simulink model "gm_untitled_vnl"  (R2022a)
settings: Solver=FixedStepDiscrete  StartTime=0.0  StopTime=2000  RelTol=1e-3
libraries: dspsigops x6, simulink x3, hdlsllib x2, simulink_need_slupdate x2
Description:
  | Symmetric FIR Filter
  | This example shows how to use HDL Coder(TM) to check, generate,
  | and verify HDL for a fixed-point symmetric FIR filter.
settings Model: Creator=okoko  LastModifiedBy=okoko
settings SolverCC: AlgebraicLoopSolver=TrustRegion
settings DataIOCC: LimitDataPoints=on  SaveOutput=off  SignalLogging=off  SaveTime=off  SignalLoggingName=logsOut
settings OptimizationCC: BlockReduction=off  BooleanDataType=off  ConditionallyExecuteInputs=off  DefaultParameterBehavior=Inlined  InlineInvariantSignals=on  ExpressionDepthLimit=2147483647  InitFltsAndDblsToZero=on  LifeSpan=inf  BufferReusableBoundary=off
settings DebuggingCC: AlgebraicLoopMsg=error  SaveWithParameterizedLinksMsg=none  UnderspecifiedInitializationDetection=Classic  MergeDetectMultiDrivingBlocksExec=none  CheckExecutionContextPreStartOutputMsg=on  SignalResolutionControl=TryResolveAllWithWarning  InheritedTsInSrcMsg=none  MultiTaskDSMMsg=warning  MultiTaskCondExecSysMsg=none  SingleTaskRateTransMsg=error  IntegerOverflowMsg=none  ParameterPrecisionLossMsg=none  FcnCallInpInsideContextMsg=warning  UnconnectedInputMsg=warning  UnconnectedOutputMsg=warning  UnconnectedLineMsg=warning  BusObjectLabelMismatch=none  AllowSymbolicDim=off  StateNameClashWarn=warning  StrictBusMsg=ErrorOnBusTreatedAsVector  SFUnexpectedBacktrackingDiag=warning  SFNoUnconditionalDefaultTransitionDiag=warning  SFExecutionAtInitializationDiag=none  SFMachineParentedDataDiag=warning  IntegerSaturationMsg=none  ArithmeticOperatorsInVariantConditions=warning
settings HardwareCC: ProdBitPerPointer=32  ProdBitPerSizeT=32  ProdBitPerPtrDiffT=32  ProdLargestAtomicFloat=None  ProdIntDivRoundTo=Undefined  ProdEndianess=Unspecified  ProdWordSize=32  ProdHWDeviceType=ASIC/FPGA->ASIC/FPGA  TargetUnknown=on  ProdEqTarget=off
settings SFSimCC: SimUseLocalCustomCode=off  CustomCodeUndefinedFunction=UseInterfaceOnly
settings RTWCC: RTWUseLocalCustomCode=off
settings CodeAppCC: StateflowObjectComments=on
settings GRTTargetCC: TargetFcnLib=ansi_tfl_tmw.mat  TargetLangStandard=C89/C90 (ANSI)  CombineOutputUpdateFcns=off  GRTInterface=on
settings ConfigComp: CovScope=ReferencedModels  CovMetricSettings=dw  CovSaveCumulativeToWorkspaceVar=on  CovSaveSingleToWorkspaceVar=on  CovExternalEMLEnable=off  CovSFcnEnable=off

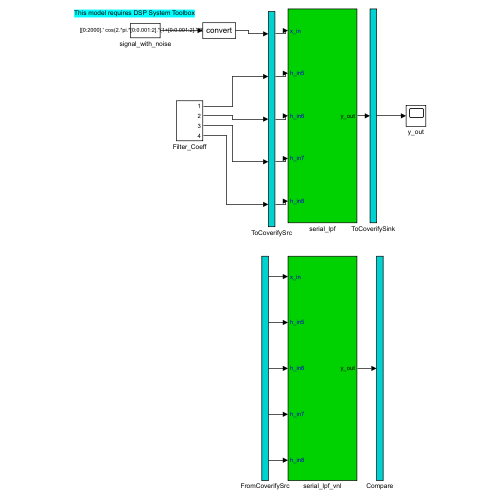
[thumbnail: Simulink's stored preview of the top-level diagram]
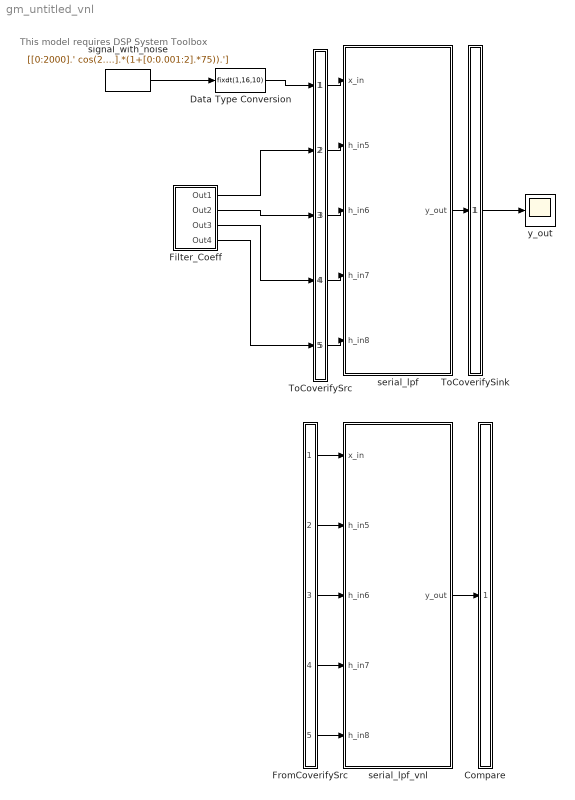
== system gm_untitled_vnl ==
  note: This model requires DSP System Toolbox
  Compare : Subsystem
      mask Display: disp('')
  Data Type Conversion : DataTypeConversion  OutDataTypeStr=fixdt(1,16,10)  SaturateOnIntegerOverflow=off  RndMeth=Floor
  Filter_Coeff : Subsystem
  FromCoverifySrc : Subsystem
      mask Display: disp('')
  ToCoverifySink : Subsystem
      mask Display: disp('')
  ToCoverifySrc : Subsystem
      mask Display: disp('')
  serial_lpf : Subsystem
  serial_lpf_vnl : Subsystem
  signal_with_noise : FromWorkspace  VariableName=[[0:2000].' cos(2.*pi.*[0:0.001:2].*(1+[0:0.001:2].*75)).']  SampleTime=1  OutputAfterFinalValue=Setting to zero
  y_out : Scope
  wires:
  signal_with_noise/1 -> Data Type Conversion/1
  ToCoverifySrc/1(out1) -> serial_lpf/1(x_in)
  ToCoverifySrc/2(out2) -> serial_lpf/2(h_in5)
  ToCoverifySrc/3(out3) -> serial_lpf/3(h_in6)
  ToCoverifySrc/4(out4) -> serial_lpf/4(h_in7)
  ToCoverifySrc/5(out5) -> serial_lpf/5(h_in8)
  serial_lpf/1(y_out) -> ToCoverifySink/1(in1)
  Data Type Conversion/1 -> ToCoverifySrc/1(in1)
  Filter_Coeff/1(Out1) -> ToCoverifySrc/2(in2)
  Filter_Coeff/2(Out2) -> ToCoverifySrc/3(in3)
  Filter_Coeff/3(Out3) -> ToCoverifySrc/4(in4)
  Filter_Coeff/4(Out4) -> ToCoverifySrc/5(in5)
  ToCoverifySink/1(out1) -> y_out/1
  FromCoverifySrc/1(out1) -> serial_lpf_vnl/1(x_in)
  FromCoverifySrc/2(out2) -> serial_lpf_vnl/2(h_in5)
  FromCoverifySrc/3(out3) -> serial_lpf_vnl/3(h_in6)
  FromCoverifySrc/4(out4) -> serial_lpf_vnl/4(h_in7)
  FromCoverifySrc/5(out5) -> serial_lpf_vnl/5(h_in8)
  serial_lpf_vnl/1(y_out) -> Compare/1(in1)

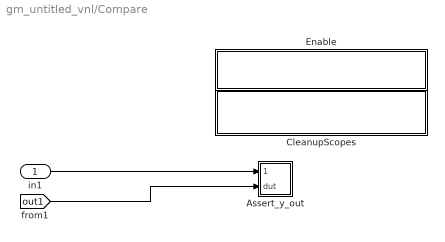
== system gm_untitled_vnl/Compare ==
  in1 : Inport
  Assert_y_out : Subsystem
  CleanupScopes : Subsystem
      settings: OpenFcn=|
      | blkName = gcb; %self block
      | idx = regexp(blkName, '/CleanupScopes$', 'once');
      | blkParent = blkName(1:idx-1);
      | blks=find_system(blkParent, 'LookUnderMasks', 'all','blocktype', 'Scope');
      | for itr = 1:length(blks)
      | 	 hScopeCfg = get_param(blks{itr},'ScopeConfiguration');
      | 	 hScopeCfg.Visible = ~ hScopeCfg.Visible;
      | end
      | drawnow;
      mask Display: fprintf(message('hdlcoder:cosim:vnl_dblclick').getString());
  Enable : Subsystem
      settings: OpenFcn=|
      | blkName = gcb;
      | idx = regexp(blkName, '/Enable$', 'once');
      | blkParent = blkName(1:idx-1);
      | blks=find_system(blkParent, 'LookUnderMasks', 'all','blocktype', 'Assertion');
      | e = get_param(blks{1}, 'Enabled');
      | if strcmp(e, 'on'), f= 'off';, else, f = 'on';, end
      | for ii=1:length(blks), set_param(blks{ii}, 'Enabled', f);, end
      | set_param(gcb, 'MaskDisplay',['fprintf(message(''hdlcoder:cosim:vnl_dblclick_assertions'',','''',upper(e),'''',').getString())']);
      mask Display: fprintf(message('hdlcoder:cosim:vnl_dblclick_assertions','OFF').getString());
  wires:
  in1/1 -> Assert_y_out/1(cosim)
  [out1] -> Assert_y_out/2(dut)

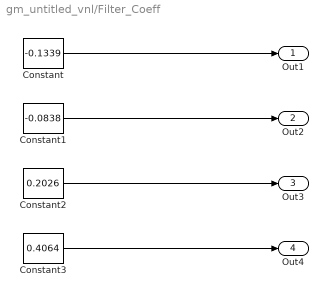
== system gm_untitled_vnl/Filter_Coeff ==
  Constant : Constant  Value=-0.1339  OutDataTypeStr=fixdt(1,16,10)  SampleTime=1
  Constant1 : Constant  Value=-0.0838  OutDataTypeStr=fixdt(1,16,10)  SampleTime=1
  Constant2 : Constant  Value=0.2026  OutDataTypeStr=fixdt(1,16,10)  SampleTime=1
  Constant3 : Constant  Value=0.4064  OutDataTypeStr=fixdt(1,16,10)  SampleTime=1
  Out1 : Outport  VectorParamsAs1DForOutWhenUnconnected=off
  Out2 : Outport  Port=2  VectorParamsAs1DForOutWhenUnconnected=off
  Out3 : Outport  Port=3  VectorParamsAs1DForOutWhenUnconnected=off
  Out4 : Outport  Port=4  VectorParamsAs1DForOutWhenUnconnected=off
  wires:
  Constant1/1 -> Out2/1
  Constant3/1 -> Out4/1
  Constant2/1 -> Out3/1
  Constant/1 -> Out1/1

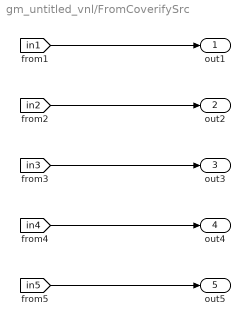
== system gm_untitled_vnl/FromCoverifySrc ==
  out1 : Outport
  out2 : Outport  Port=2
  out3 : Outport  Port=3
  out4 : Outport  Port=4
  out5 : Outport  Port=5
  wires:
  [in1] -> out1/1
  [in2] -> out2/1
  [in3] -> out3/1
  [in4] -> out4/1
  [in5] -> out5/1

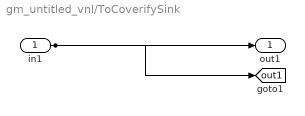
== system gm_untitled_vnl/ToCoverifySink ==
  in1 : Inport
  out1 : Outport
  tag scope: out1=global
  wires:
  in1/1 -> out1/1, [out1]

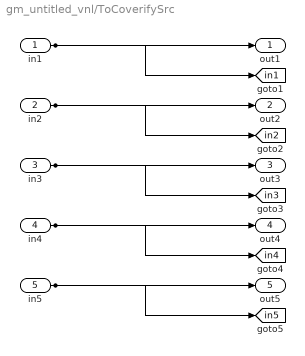
== system gm_untitled_vnl/ToCoverifySrc ==
  in1 : Inport
  in2 : Inport  Port=2
  in3 : Inport  Port=3
  in4 : Inport  Port=4
  in5 : Inport  Port=5
  out1 : Outport
  out2 : Outport  Port=2
  out3 : Outport  Port=3
  out4 : Outport  Port=4
  out5 : Outport  Port=5
  tag scope: in1=global, in2=global, in3=global, in4=global, in5=global
  wires:
  in1/1 -> out1/1, [in1]
  in2/1 -> out2/1, [in2]
  in3/1 -> out3/1, [in3]
  in4/1 -> out4/1, [in4]
  in5/1 -> out5/1, [in5]

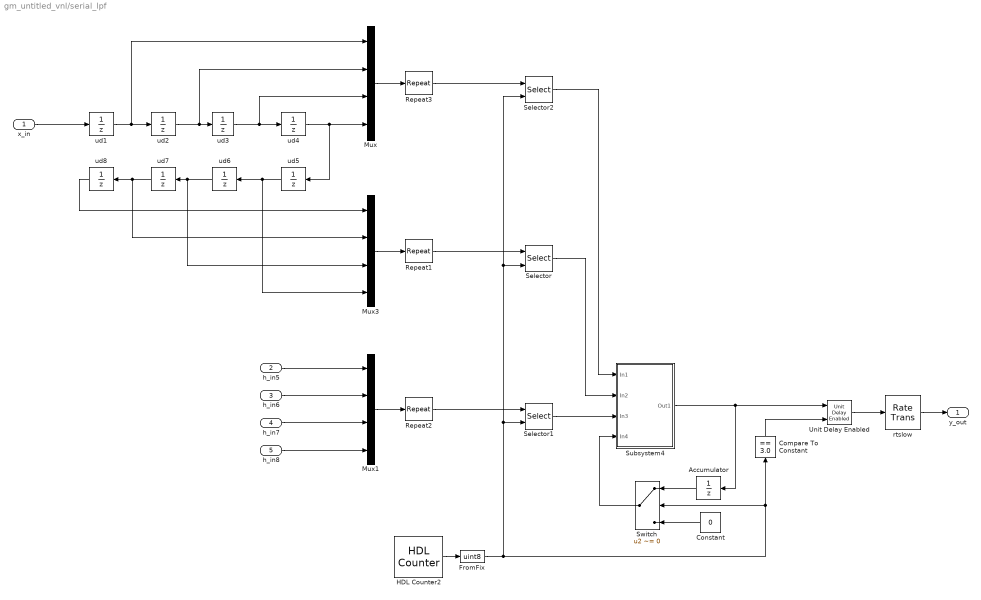
== system gm_untitled_vnl/serial_lpf ==
  x_in : Inport  SampleTime=1
  h_in5 : Inport  Port=2
  h_in6 : Inport  Port=3
  h_in7 : Inport  Port=4
  h_in8 : Inport  Port=5
  Accumulator : UnitDelay  SampleTime=-1  HasFrameUpgradeWarning=on
  Compare To Constant : simulink/Logic and Bit Operations/Compare To Constant  relop===  const=3.0  OutDataTypeStr=boolean
  Constant : Constant  Value=0  OutDataTypeStr=Inherit: Inherit via back propagation  SampleTime=-1
  FromFix : DataTypeConversion  OutDataTypeStr=uint8  SaturateOnIntegerOverflow=off  RndMeth=Floor
  HDL Counter2 : hdlsllib/Sources/HDL Counter  CountType=Count limited  CountInit=0  CountStep=1  CountMax=3  CountFromType=Initial value  CountFrom=0  CountResetPort=off  CountLoadPort=off  CountEnbPort=off  CountDirPort=off  CountHitOutputPort=off  CountDataType=Unsigned  CountWordLen=2  CountFracLen=0  CountSampTime=-1
  Mux : Mux
  Mux1 : Mux
  Mux3 : Mux
  Repeat1 : dspsigops/Repeat  N=4  RateOptions=Allow multirate processing  ic=0  mode=Unused parameter value
  Repeat2 : dspsigops/Repeat  N=4  RateOptions=Allow multirate processing  ic=0  mode=Unused parameter value
  Repeat3 : dspsigops/Repeat  N=4  RateOptions=Allow multirate processing  ic=0  mode=Unused parameter value
  Selector : Selector  IndexMode=Zero-based  InputPortWidth=4  IndexOptions=Index vector (port)  Indices=[1 3]  OutputSizes=1
  Selector1 : Selector  IndexMode=Zero-based  InputPortWidth=4  IndexOptions=Index vector (port)  Indices=[1 3]  OutputSizes=1
  Selector2 : Selector  IndexMode=Zero-based  InputPortWidth=4  IndexOptions=Index vector (port)  Indices=[1 3]  OutputSizes=1
  Subsystem4 : Subsystem  TreatAsAtomicUnit=on
  Switch : Switch  Criteria=u2 ~= 0  OutDataTypeStr=fixdt(1,35,20)  SaturateOnIntegerOverflow=off  InputSameDT=off
  Unit Delay Enabled : simulink_need_slupdate/Unit Delay Enabled  vinit=0.0  tsamp=-1
      settings: SourceProductBaseCode=SL
  rtslow : RateTransition
  ud{1..8} (8 alike) : UnitDelay  SampleTime=-1  HasFrameUpgradeWarning=on
  y_out : Outport  SampleTime=1  VectorParamsAs1DForOutWhenUnconnected=off
  wires:
  Selector/1 -> Subsystem4/2(In2)
  Mux/1 -> Repeat3/1
  Repeat1/1 -> Selector/1
  Subsystem4/1(Out1) -> Accumulator/1, Unit Delay Enabled/1
  x_in/1 -> ud1/1
  ud7/1 -> Mux3/2, ud8/1
  h_in5/1 -> Mux1/1
  h_in6/1 -> Mux1/2
  h_in7/1 -> Mux1/3
  h_in8/1 -> Mux1/4
  HDL Counter2/1 -> FromFix/1
  Mux1/1 -> Repeat2/1
  Selector1/1 -> Subsystem4/3(In3)
  Selector2/1 -> Subsystem4/1(In1)
  Mux3/1 -> Repeat1/1
  Repeat3/1 -> Selector2/1
  Repeat2/1 -> Selector1/1
  rtslow/1 -> y_out/1
  Unit Delay Enabled/1 -> rtslow/1
  Accumulator/1 -> Switch/1
  Constant/1 -> Switch/3
  Switch/1 -> Subsystem4/4(In4)
  Compare To Constant/1 -> Unit Delay Enabled/2
  ud1/1 -> Mux/1, ud2/1
  ud2/1 -> Mux/2, ud3/1
  ud3/1 -> Mux/3, ud4/1
  ud4/1 -> Mux/4, ud5/1
  ud5/1 -> Mux3/4, ud6/1
  ud6/1 -> Mux3/3, ud7/1
  ud8/1 -> Mux3/1
  FromFix/1 -> Selector1/2, Selector/2, Selector2/2, Switch/2, Compare To Constant/1

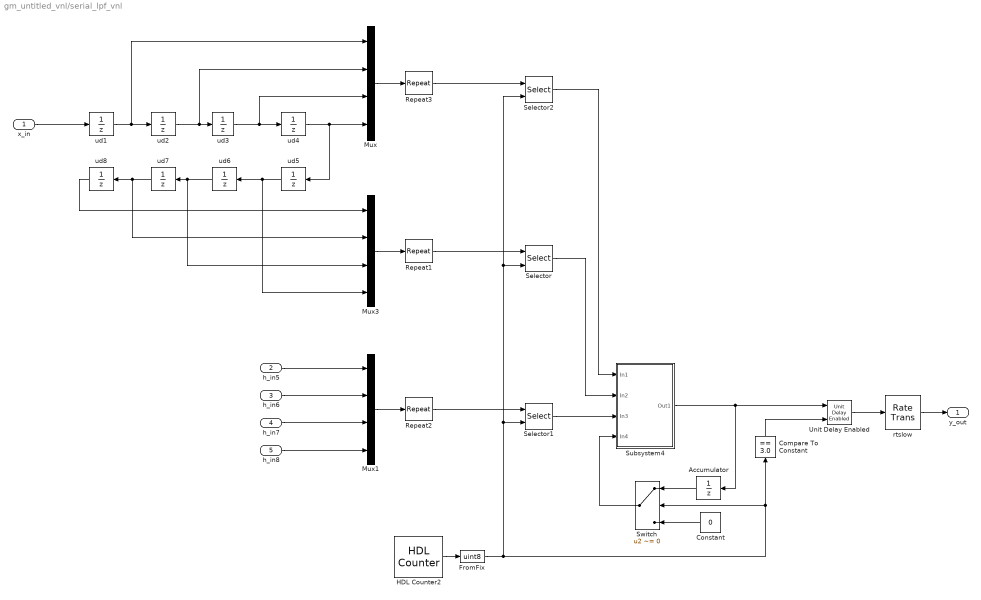
== system gm_untitled_vnl/serial_lpf_vnl ==
  x_in : Inport  SampleTime=1
  h_in5 : Inport  Port=2
  h_in6 : Inport  Port=3
  h_in7 : Inport  Port=4
  h_in8 : Inport  Port=5
  Accumulator : UnitDelay  SampleTime=-1  HasFrameUpgradeWarning=on
  Compare To Constant : simulink/Logic and Bit Operations/Compare To Constant  relop===  const=3.0  OutDataTypeStr=boolean
  Constant : Constant  Value=0  OutDataTypeStr=Inherit: Inherit via back propagation  SampleTime=-1
  FromFix : DataTypeConversion  OutDataTypeStr=uint8  SaturateOnIntegerOverflow=off  RndMeth=Floor
  HDL Counter2 : hdlsllib/Sources/HDL Counter  CountType=Count limited  CountInit=0  CountStep=1  CountMax=3  CountFromType=Initial value  CountFrom=0  CountResetPort=off  CountLoadPort=off  CountEnbPort=off  CountDirPort=off  CountHitOutputPort=off  CountDataType=Unsigned  CountWordLen=2  CountFracLen=0  CountSampTime=-1
  Mux : Mux
  Mux1 : Mux
  Mux3 : Mux
  Repeat1 : dspsigops/Repeat  N=4  RateOptions=Allow multirate processing  ic=0  mode=Unused parameter value
  Repeat2 : dspsigops/Repeat  N=4  RateOptions=Allow multirate processing  ic=0  mode=Unused parameter value
  Repeat3 : dspsigops/Repeat  N=4  RateOptions=Allow multirate processing  ic=0  mode=Unused parameter value
  Selector : Selector  IndexMode=Zero-based  InputPortWidth=4  IndexOptions=Index vector (port)  Indices=[1 3]  OutputSizes=1
  Selector1 : Selector  IndexMode=Zero-based  InputPortWidth=4  IndexOptions=Index vector (port)  Indices=[1 3]  OutputSizes=1
  Selector2 : Selector  IndexMode=Zero-based  InputPortWidth=4  IndexOptions=Index vector (port)  Indices=[1 3]  OutputSizes=1
  Subsystem4 : Subsystem  TreatAsAtomicUnit=on
  Switch : Switch  Criteria=u2 ~= 0  OutDataTypeStr=fixdt(1,35,20)  SaturateOnIntegerOverflow=off  InputSameDT=off
  Unit Delay Enabled : simulink_need_slupdate/Unit Delay Enabled  vinit=0.0  tsamp=-1
      settings: SourceProductBaseCode=SL
  rtslow : RateTransition
  ud{1..8} (8 alike) : UnitDelay  SampleTime=-1  HasFrameUpgradeWarning=on
  y_out : Outport  SampleTime=1  VectorParamsAs1DForOutWhenUnconnected=off
  wires:
  FromFix/1 -> Compare To Constant/1, Switch/2, Selector2/2, Selector/2, Selector1/2
  ud8/1 -> Mux3/1
  ud6/1 -> ud7/1, Mux3/3
  ud5/1 -> ud6/1, Mux3/4
  ud4/1 -> ud5/1, Mux/4
  ud3/1 -> ud4/1, Mux/3
  ud2/1 -> ud3/1, Mux/2
  ud1/1 -> ud2/1, Mux/1
  Compare To Constant/1 -> Unit Delay Enabled/2
  Switch/1 -> Subsystem4/4(In4)
  Constant/1 -> Switch/3
  Accumulator/1 -> Switch/1
  Unit Delay Enabled/1 -> rtslow/1
  rtslow/1 -> y_out/1
  Repeat2/1 -> Selector1/1
  Repeat3/1 -> Selector2/1
  Mux3/1 -> Repeat1/1
  Selector2/1 -> Subsystem4/1(In1)
  Selector1/1 -> Subsystem4/3(In3)
  Mux1/1 -> Repeat2/1
  HDL Counter2/1 -> FromFix/1
  h_in8/1 -> Mux1/4
  h_in7/1 -> Mux1/3
  h_in6/1 -> Mux1/2
  h_in5/1 -> Mux1/1
  ud7/1 -> ud8/1, Mux3/2
  x_in/1 -> ud1/1
  Subsystem4/1(Out1) -> Unit Delay Enabled/1, Accumulator/1
  Repeat1/1 -> Selector/1
  Mux/1 -> Repeat3/1
  Selector/1 -> Subsystem4/2(In2)

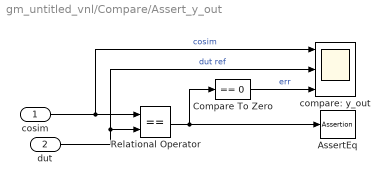
== system gm_untitled_vnl/Compare/Assert_y_out ==
  cosim : Inport
  dut : Inport  Port=2
  AssertEq : Assertion  StopWhenAssertionFail=off
  Compare To Zero : simulink/Logic and Bit Operations/Compare To Zero  relop===  OutDataTypeStr=boolean
  Relational Operator : RelationalOperator  Operator===  OutDataTypeStr=boolean  InputSameDT=off
  compare: y_out : Scope  NumInputPorts=3
  wires:
  Compare To Zero/1 -> compare: y_out/3  "err"
  Relational Operator/1 -> Compare To Zero/1, AssertEq/1
  cosim/1 -> compare: y_out/1, Relational Operator/1  "cosim"
  dut/1 -> compare: y_out/2, Relational Operator/2  "dut ref"

== system gm_untitled_vnl/Compare/CleanupScopes ==

== system gm_untitled_vnl/Compare/Enable ==

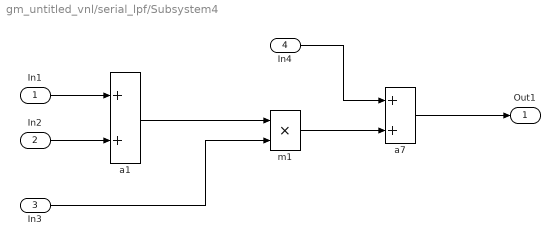
== system gm_untitled_vnl/serial_lpf/Subsystem4 ==
  In1 : Inport
  In2 : Inport  Port=2
  In3 : Inport  Port=3
  In4 : Inport  Port=4
  a1 : Sum
  a7 : Sum
  m1 : Product  RndMeth=Zero
  Out1 : Outport  OutDataTypeStr=fixdt(1,35,20)  SampleTime=0.25  VectorParamsAs1DForOutWhenUnconnected=off
  wires:
  a1/1 -> m1/1
  a7/1 -> Out1/1
  In1/1 -> a1/1
  In2/1 -> a1/2
  In3/1 -> m1/2
  In4/1 -> a7/1
  m1/1 -> a7/2

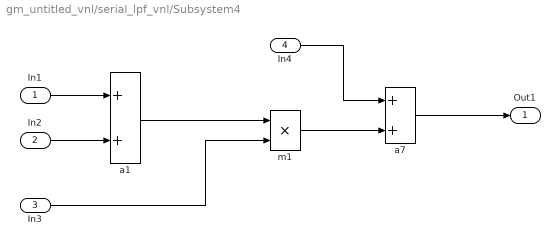
== system gm_untitled_vnl/serial_lpf_vnl/Subsystem4 ==
  In1 : Inport
  In2 : Inport  Port=2
  In3 : Inport  Port=3
  In4 : Inport  Port=4
  a1 : Sum
  a7 : Sum
  m1 : Product  RndMeth=Zero
  Out1 : Outport  OutDataTypeStr=fixdt(1,35,20)  SampleTime=0.25  VectorParamsAs1DForOutWhenUnconnected=off
  wires:
  m1/1 -> a7/2
  In4/1 -> a7/1
  In3/1 -> m1/2
  In2/1 -> a1/2
  In1/1 -> a1/1
  a7/1 -> Out1/1
  a1/1 -> m1/1
